simulink model "simpowersystems_constant_power"  (Simulink 8.1)
settings: Solver=FixedStepDiscrete  StartTime=0.0  StopTime=inf  FixedStep=1  MaxStep=1/60  RelTol=1e-3
InitFcn:
  | Ts = 1e-5;
libraries: powerlib x4, simulink x2, powerlib_extras x1, CampusEnergyModeling x1
settings Model: Creator=sfrank1  LastModifiedBy=sfrank1

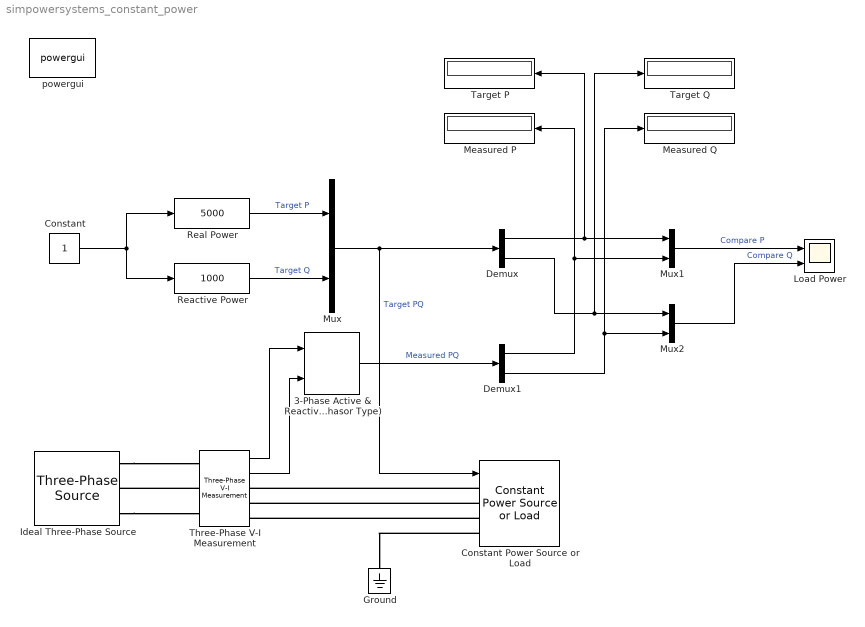
== system simpowersystems_constant_power ==
  3-Phase Active & Reactive Power (Phasor Type) : powerlib_extras/Phasor Library/3-Phase Active & Reactive Power (Phasor Type)
  Constant : Constant
  Constant Power Source or Load : CampusEnergyModeling/Electrical/Constant Power Source or Load  Conven=load  PNom=10000  QNom=0  VNom=480  fNom=60  VLow=0.7
  Demux : Demux  Outputs=2
  Demux1 : Demux  Outputs=2
  Ground : powerlib/Elements/Ground  LConnTagsString=a
  Ideal Three-Phase Source : powerlib/Electrical Sources/Three-Phase Source  Voltage=480  PhaseAngle=0  Frequency=60  InternalConnection=Yg  SpecifyImpedance=on  Resistance=0  Inductance=0  ShortCircuitLevel=1e6  BaseVoltage=480  XRratio=1  BusType=swing  Pref=0  Qref=0  Qmin=-inf  Qmax=inf
  Load Power : Scope  NumInputPorts=2
      settings: TickLabels=on  YMin=-3000~0  YMax=3000~5.5e-13
  Measured P : Display
  Measured Q : Display
  Mux : Mux  Inputs=2
  Mux1 : Mux  Inputs=2
  Mux2 : Mux  Inputs=2
  Reactive Power : simulink/Math Operations/Slider Gain  low=-5000  gain=1000  high=5000
  Real Power : simulink/Math Operations/Slider Gain  low=-5000  gain=5000  high=10000
  Target P : Display
  Target Q : Display
  Three-Phase V-I Measurement : powerlib/Measurements/Three-Phase V-I Measurement  VoltageMeasurement=phase-to-ground  SetLabelV=off  LabelV=Vabc  Vpu=off  VpuLL=off  CurrentMeasurement=yes  SetLabelI=off  LabelI=Iabc  Ipu=off  Pbase=100e6  Vbase=500e3  OutputType=Complex  PhasorSimulation=on  PSBequivalent=0
  powergui : powerlib/powergui  Priority=1  SimulationMode=Phasor  SolverType=Tustin  SampleTime=50e-6  frequency=60  SPID=off  DisableSnubberDevices=off  DisableRonSwitches=off  DisableVfSwitches=off  SwTol=0  Interpol=off  DisplayEquations=off  frequencyindice=60  Pbase=100e3  ErrMax=1e-4  Iterations=50  UnitsV=kV  UnitsW=MW  FunctionMessages=off  echomessages=off  HookPort=off  EnableUseOfTLC=off  x0status=blocks  RestoreLinks=warning  ResistiveCurrentMeasurement=off  Frange=[0:2:500]  Ylog=off  Xlog=on  ShowGrid=off  save=off  variable=ZData  ZoomFFT=off  StartTime=0.0  cycles=1  DisplayStyle=1  fundamental=60  FreqAxis=off  MaxFrequency=1000  frequencyindicesteady=1  RmsSteady=1  display=off  Ts=0  methode=off
  wires:
  Constant/1 -> Reactive Power/1, Real Power/1
  Real Power/1 -> Mux/1  "Target P"
  Mux/1 -> Constant Power Source or Load/1, Demux/1  "Target PQ"
  Reactive Power/1 -> Mux/2  "Target Q"
  3-Phase Active & Reactive Power (Phasor Type)/1 -> Demux1/1  "Measured PQ"
  Mux1/1 -> Load Power/1  "Compare P"
  Mux2/1 -> Load Power/2  "Compare Q"
  Demux/1 -> Mux1/1, Target P/1
  Demux1/1 -> Measured P/1, Mux1/2
  Demux/2 -> Mux2/1, Target Q/1
  Demux1/2 -> Mux2/2, Measured Q/1
  Three-Phase V-I Measurement/2 -> 3-Phase Active & Reactive Power (Phasor Type)/2
  Three-Phase V-I Measurement/1 -> 3-Phase Active & Reactive Power (Phasor Type)/1
  connections:
  Constant Power Source or Load/LConn4 -- Ground/LConn1
  Ideal Three-Phase Source/RConn1 -- Three-Phase V-I Measurement/LConn1
  Three-Phase V-I Measurement/LConn2 -- Ideal Three-Phase Source/RConn2
  Ideal Three-Phase Source/RConn3 -- Three-Phase V-I Measurement/LConn3
  Constant Power Source or Load/LConn1 -- Three-Phase V-I Measurement/RConn1
  Constant Power Source or Load/LConn2 -- Three-Phase V-I Measurement/RConn2
  Constant Power Source or Load/LConn3 -- Three-Phase V-I Measurement/RConn3
